simulink model "ball_bounce"  (R2019b)
settings: Solver=ode15s  StartTime=0.0  StopTime=8  MaxStep=.1  RelTol=1e-6  EnableMultiTasking=on
values from neighbouring files (symbols this model uses):
  x0 = 15.0    (= 15)    [reach.m]    (also in reach_magic.m = [x01;x02]; reach_pos.m = 24; reach_pos_gen.m)
undefined symbols (not defined in the file or in its folder): v0
settings Model: ExtModeAutoUpdateStatusClock=off  Creator=The MathWorks, Inc.  LastModifiedBy=manzand
settings SolverCC: ConsecutiveZCsStepRelTol=1*128*eps  ZeroCrossControl=EnableAll
settings DataIOCC: SaveFormat=StructureWithTime  ReturnWorkspaceOutputs=off
settings OptimizationCC: ExpressionDepthLimit=2147483647  InitFltsAndDblsToZero=on  EfficientMapNaN2IntZero=off  LifeSpan=inf
settings DebuggingCC: UnderspecifiedInitializationDetection=Classic  MergeDetectMultiDrivingBlocksExec=none  SignalResolutionControl=TryResolveAllWithWarning  SolverPrmCheckMsg=warning  FcnCallInpInsideContextMsg=warning  StateNameClashWarn=warning  PregeneratedLibrarySubsystemCodeDiagnostic=none  SFUnexpectedBacktrackingDiag=warning  SFNoUnconditionalDefaultTransitionDiag=warning  SFExecutionAtInitializationDiag=none  ArithmeticOperatorsInVariantConditions=warning
settings HardwareCC: ProdBitPerPointer=32  ProdBitPerSizeT=32  ProdBitPerPtrDiffT=32  ProdLargestAtomicFloat=None  ProdIntDivRoundTo=Undefined  ProdEndianess=Unspecified  ProdWordSize=32  ProdHWDeviceType=32-bit Generic  TargetBitPerLong=64  TargetBitPerPointer=64  TargetBitPerSizeT=64  TargetBitPerPtrDiffT=64  TargetLongLongMode=on  TargetIntDivRoundTo=Zero  TargetEndianess=LittleEndian  TargetWordSize=64  TargetHWDeviceType=MATLAB Host
settings ModelReferenceCC: PropagateSignalLabelsOutOfModel=off
settings SFSimCC: SFSimEcho=off  SimUseLocalCustomCode=off  SimParseCustomCode=off  CustomCodeUndefinedFunction=UseInterfaceOnly
settings RTWCC: Description=Generic Real-Time Target  RTWUseLocalCustomCode=off
settings CodeAppCC: StateflowObjectComments=on
settings GRTTargetCC: TargetLangStandard=C89/C90 (ANSI)  GeneratePreprocessorConditionals=Disable all  CombineOutputUpdateFcns=off  GRTInterface=on
settings ConfigComp: CovMetricSettings=dw  CovHtmlReporting=on  CovSaveCumulativeToWorkspaceVar=on  CovSaveSingleToWorkspaceVar=on  CovExternalEMLEnable=off  CovSFcnEnable=off

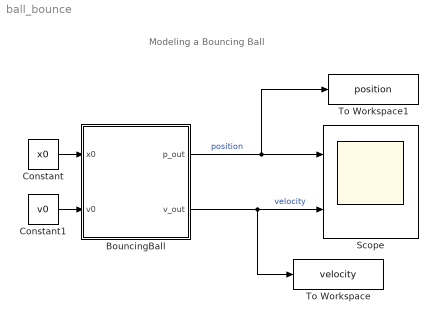
== system ball_bounce ==
  note: Modeling a Bouncing Ball
  BouncingBall : Stateflow chart  TreatAsAtomicUnit=on
  Constant : Constant  Value=x0
  Constant1 : Constant  Value=v0
  Scope : Scope  NumInputPorts=2
  To Workspace : ToWorkspace  VariableName=velocity  SaveFormat=Structure With Time  SampleTime=-1
  To Workspace1 : ToWorkspace  VariableName=position  SaveFormat=Structure With Time  SampleTime=-1
  wires:
  BouncingBall/1(p_out) -> To Workspace1/1, Scope/1  "position"
  BouncingBall/2(v_out) -> To Workspace/1, Scope/2  "velocity"
  Constant/1 -> BouncingBall/1(x0)
  Constant1/1 -> BouncingBall/2(v0)

== stateflow chart ball_bounce/BouncingBall ==
  settings: updateMethod=CONTINUOUS  executeAtInitialization=1  initializeOutput=1
  state Falling
    du:
    % derivatives
    p_dot = v;
    v_dot = -9.81;
    % outputs
    p_out = p;
    v_out = v;
  (default) -> Falling : {
      | p = x0;
      | v = v0;
      | }
  Falling -> Falling : [ p <= 0  && v < 0 ]
      | {
      | p = 0;
      | v = -0.8.*v;
      | }
  data: p_out output double size=1; p local double; v local double; v_out output double size=1; x0 input double; v0 input double
  data p settings: updateMethod=SF_CONTINUOUS_TIME_DATA
  data v settings: updateMethod=SF_CONTINUOUS_TIME_DATA
